simulink model "Test_Tricopter_Model"  (R2015a)
settings: Solver=ode3  SolverMode=SingleTasking  StartTime=0.0  StopTime=20  FixedStep=T_sim  RelTol=1e-3
PreLoadFcn:
  | LoadLibraries
values from neighbouring files (symbols this model uses):
  a = 10.26    [SetupComplete.m]
  A_x = 0.015    [SetupComplete.m]
  A_y = A_x    (= 0.015)    [SetupComplete.m]
  A_z = 0.16    [SetupComplete.m]
  C_d0 = 0.001193    [SetupComplete.m]
  C_x = 1.2    [SetupComplete.m]
  C_y = C_x    (= 1.2)    [SetupComplete.m]
  C_z = 2.2    [SetupComplete.m]
  CG_0 = [0,0,0.02]'    [SetupComplete.m]
  g = 9.81    [SetupComplete.m]
  h = 0.08    [SetupComplete.m]
  h_FA = 0.02    [SetupComplete.m]
  h_M = 0.064    [SetupComplete.m]
  I_BAC_0 = [ Ix,0,Ixz;0,Iy,0;Ixz,0,Iz]    [SetupComplete.m]
  I_prop = 1/4*M_eq*R^2*diag([1,1,2])    [SetupComplete.m]
  I_tube = [1/2*M_tube*R_tube_eq^2,0,  0  ;           0 ,1/3*M_tube*l_arm^2,0;             0  ,0,1/3*M_tube*l_arm^2]    [SetupComplete.m]
  Initial_Omegas = [1;1;1]*Omega_hover    [Run3Copter.m]
  J_FA = I_prop(1,1) + m_prop*h^2  + m_FA*h_FA^2 + m_M*h_M^2    [SetupComplete.m]
  J_T = J_m+1/2*M_eq*R^2    (= 2.000642e-05)    [SetupComplete.m]
  Ki = lqi(LM_4DOF_aug, Q,R)    [robust_controller.m]
  l = 0.3450    (= 0.345)    [NDI_components.m]    (also in SetupComplete.m; robust_controller.m)
  l_arm = 0.264    [SetupComplete.m]
  m = 3.51    [SetupComplete.m]
  m_0 = 2.61    [SetupComplete.m]
  m_FA = 0.02    [SetupComplete.m]
  m_M = 0.300    (= 0.3)    [SetupComplete.m]
  m_prop = 0.02    [SetupComplete.m]
  R = 0.1778    [SetupComplete.m]    (also in robust_controller.m = eye(4))
  rho = 1.15    [SetupComplete.m]
  sigma = b*c/(pi*R)    (= 0.107416159567)    [SetupComplete.m]
  T_sim = 0.01    [Run3Copter.m]
  theta_0 = 0.38397    [SetupComplete.m]
  theta_1 = -0.2967    [SetupComplete.m]
  trim_simplemodel = [0.589627915568 -2.20656039197 0 0.588313336084 0 0 0.588313330414 0 0]    [trimvalues.mat]
  V_4DOF_last = [0.0122475086001 0.00870447045314 -0.0292257707267 -0.0198753669721 -0.00290766514824 -0.0269511839788 0.0344308792695 -0.0305235710433 -0.0274078219028 -0.0329291952852 -0.0272335702183 -0.00643013158961 ... (1500 elements, 50x30)]    [NN_c_weights.mat]
  v_i0 = sqrt( 1/3*m*g/(2*rho*pi*R^2)  )    [SetupComplete.m]
  W_4DOF_last = [0.0132359246225 -0.0402459595001 -0.0221501781133 0.0046881519205 0.0457506835434 0.0464888535199 -0.0342386918322 0.0470592781761 0.0457166948243 -0.00146243512772 0.0300280468889 -0.0358113661373 ... (204 elements, 4x51)]    [NN_c_weights.mat]
undefined symbols (not defined in the file or in its folder): DOWN_0, EAST_0, Motor, NORTH_0, P_0, Prop, Q_0, R_0, sigmatest, U_0, V_0, v_i_adim, Vx_adim, Vz_adim, W_0
undefined symbols (not defined in the file): Initial_Torques, Rotation_sign, Tau_motors
libraries: simulink x61, XXCopter x32, vrlib x26, simulink_extras x6, aerolib6dofsys x3, qcatlib x3, dspinverses x3, lib_controller x2, aerolibtransform2 x2, aerolib6dof2 x1
(part 5 of 10)

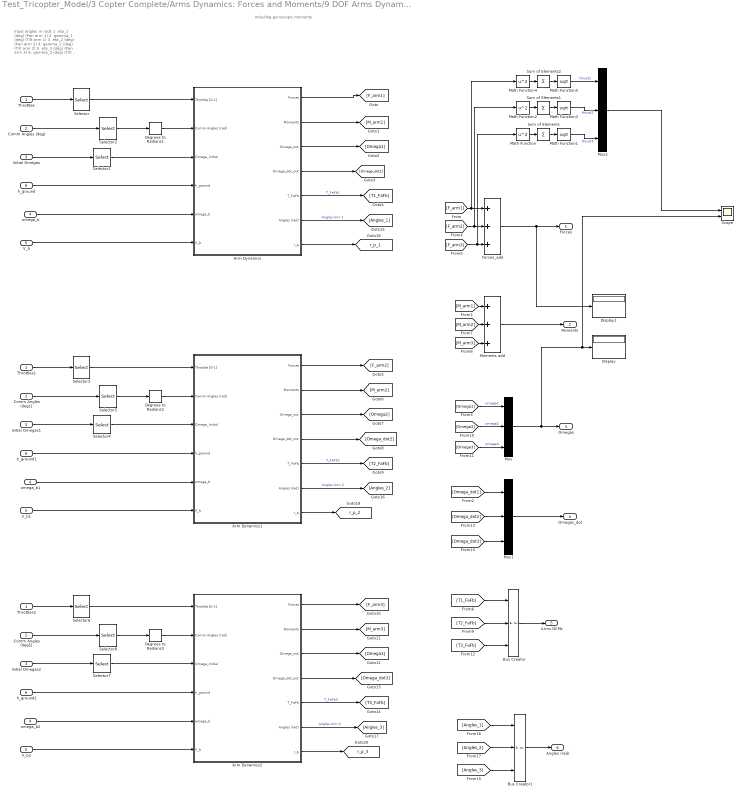
== system Test_Tricopter_Model/3 Copter Complete/Arms Dynamics: Forces and Moments/9 DOF Arms Dynamics: Forces and Moments/9 DOF Arms Dynamics: Forces and Moments ==
  note: Including gyroscopic moments
  note: Input angles in rads
      |
      | 1. eta_1 (deg)  (Pan arm 1)
      | 2. gamma_1 (deg)  (Tilt arm 1)
      |
      | 3. eta_2 (deg)  (Pan arm 2)
      | 4. gamma_2 (deg)  (Tilt arm 2)
      |
      | 5. eta_3 (deg)  (Pan arm  3)
      | 6. gamma_3 (deg)  (Tilt arm 3)
  Throttles : Inport
  Comm Angles (deg) : Inport  Port=2
  Initial Omegas : Inport  Port=3
  omega_b : Inport  Port=4
  V_b : Inport  Port=5
  h_ground : Inport  Port=6
  Arm Dynamics : Subsystem  TreatAsAtomicUnit=on  mask(Arm dynamics, kinematics, forces and moments){Rot_sign=Rotation_sign(1), tau=Tau_motors, arm_hub_pos=l*[1;0;0], arm_axis=[l_arm;0;0], arm_num=1, eta_dir=[1;0;0], gamma_dir=[0;1;0], J_T=J_T, J_FA=J_FA, h=h, Torq_ini=Initial_Torques(1), Omega_ini=Initial_Omegas(1), init_eta=0, init_gamma=0, omega_n=35, xi=1.45, c=0}
      mask prompts: Rot_sign "Rotation sign"; tau "Tau motors"; arm_hub_pos "Arm Hub position"; arm_axis "Arm Hub from servo"; arm_num "Arm number"; eta_dir "eta direcction"; gamma_dir "gamma direction"; J_T "Inertia Motor+prop"; J_FA "Inertia Forearm"; h "h propeller hub"; Torq_ini "Torque Initial Condition"; Omega_ini "Omega Initial Condition"; init_eta "Initial eta  (rad)"; init_gamma "Initial gamma  (rad)"; omega_n "Servo natural frequency"; xi "Servo damping"; c "Derivative param"
      mask help:
      | This block only accepts arms oriented in x-axis or y-axis: eta and gamma directions can only be [1,0,0] or [0,1,0]
      | Note rotations order is [eta (pan) ,gamma (tilt),0]
      |
      | If Arm number 1 (Forward one)
      | eta_dir=[1,0,0]
      | gamma_dir=[0,1,0]
      |
      | If Arm number 2 or 3 (rear ones)
      | eta_dir=[0,1,0]
      | gamma_dir=[1,0,0]
      mask TypeOptions Rot_sign: Aerodynamics Propeller/Rot_sign | Gyroscopic Moments/Rot_sign
      mask TypeOptions tau: ESC+Motor Dynamcis/tau
      mask TypeOptions arm_hub_pos: Arms Kinematics/Arm_hub_position
      mask TypeOptions arm_axis: Gyroscopic Moments/Arm_axis
      mask TypeOptions arm_num: Arms Kinematics/Arm_number
      mask TypeOptions eta_dir: Arms Kinematics/eta_dir | Gyroscopic Moments/eta_dir
      mask TypeOptions gamma_dir: Arms Kinematics/gamma_dir | Gyroscopic Moments/gamma_dir
      mask TypeOptions J_T: ESC+Motor Dynamcis/J_T | Gyroscopic Moments/J_T
      mask TypeOptions J_FA: Gyroscopic Moments/J_FA
      mask TypeOptions h: Arms Kinematics/h_prop
      mask TypeOptions Torq_ini: Initial_torque/X0
      mask TypeOptions Omega_ini: initial_omega/X0
      mask TypeOptions init_eta: Servos Dynamics/init_eta
      mask TypeOptions omega_n: Servos Dynamics/omega_n
      mask TypeOptions xi: Servos Dynamics/xi
      mask TypeOptions c: Servos Dynamics/derv_param
      mask Display:
      | % fprintf(' Arm number %i \n dynamics',arm_num)
      | 
      | 
      | disp(['{\bf \fontsize{16}',sprintf('Arm number\n\n'),num2str(arm_num),sprintf('\n\n Dynamics '),'}'], 'texmode','on');
  Arm Dynamics1 : Subsystem  TreatAsAtomicUnit=on  mask(Arm dynamics, kinematics, forces and moments){Rot_sign=Rotation_sign(2), tau=Tau_motors, arm_hub_pos=l*[-1/2;sqrt(3)/2;0], arm_axis=[0;l_arm;0], arm_num=2, eta_dir=[0;1;0], gamma_dir=[1;0;0], J_T=J_T, J_FA=J_FA, h=h, Torq_ini=Initial_Torques(2), Omega_ini=Initial_Omegas(2), init_eta=0, init_gamma=0, omega_n=35, xi=1.45, c=0}
      mask prompts: Rot_sign "Rotation sign"; tau "Tau motors"; arm_hub_pos "Arm Hub position"; arm_axis "Arm Hub from servo"; arm_num "Arm number"; eta_dir "eta direcction"; gamma_dir "gamma direction"; J_T "Inertia Motor+prop"; J_FA "Inertia Forearm"; h "h propeller hub"; Torq_ini "Torque Initial Condition"; Omega_ini "Omega Initial Condition"; init_eta "Initial eta  (rad)"; init_gamma "Initial gamma  (rad)"; omega_n "Servo natural frequency"; xi "Servo damping"; c "Derivative param"
      mask help:
      | This block only accepts arms oriented in x-axis or y-axis: eta and gamma directions can only be [1,0,0] or [0,1,0]
      | Note rotations order is [eta (pan) ,gamma (tilt),0]
      |
      | If Arm number 1 (Forward one)
      | eta_dir=[1,0,0]
      | gamma_dir=[0,1,0]
      |
      | If Arm number 2 or 3 (rear ones)
      | eta_dir=[0,1,0]
      | gamma_dir=[1,0,0]
      mask TypeOptions Rot_sign: Aerodynamics Propeller/Rot_sign | Gyroscopic Moments/Rot_sign
      mask TypeOptions tau: ESC+Motor Dynamcis/tau
      mask TypeOptions arm_hub_pos: Arms Kinematics/Arm_hub_position
      mask TypeOptions arm_axis: Gyroscopic Moments/Arm_axis
      mask TypeOptions arm_num: Arms Kinematics/Arm_number
      mask TypeOptions eta_dir: Arms Kinematics/eta_dir | Gyroscopic Moments/eta_dir
      mask TypeOptions gamma_dir: Arms Kinematics/gamma_dir | Gyroscopic Moments/gamma_dir
      mask TypeOptions J_T: ESC+Motor Dynamcis/J_T | Gyroscopic Moments/J_T
      mask TypeOptions J_FA: Gyroscopic Moments/J_FA
      mask TypeOptions h: Arms Kinematics/h_prop
      mask TypeOptions Torq_ini: Initial_torque/X0
      mask TypeOptions Omega_ini: initial_omega/X0
      mask TypeOptions init_eta: Servos Dynamics/init_eta
      mask TypeOptions omega_n: Servos Dynamics/omega_n
      mask TypeOptions xi: Servos Dynamics/xi
      mask TypeOptions c: Servos Dynamics/derv_param
      mask Display:
      | % fprintf(' Arm number %i \n dynamics',arm_num)
      | 
      | 
      | disp(['{\bf \fontsize{16}',sprintf('Arm number\n\n'),num2str(arm_num),sprintf('\n\n Dynamics '),'}'], 'texmode','on');
  Arm Dynamics2 : Subsystem  TreatAsAtomicUnit=on  mask(Arm dynamics, kinematics, forces and moments){Rot_sign=Rotation_sign(3), tau=Tau_motors, arm_hub_pos=l*[-1/2;-sqrt(3)/2;0], arm_axis=[0;-l_arm;0], arm_num=3, eta_dir=[0;1;0], gamma_dir=[1;0;0], J_T=J_T, J_FA=J_FA, h=h, Torq_ini=Initial_Torques(3), Omega_ini=Initial_Omegas(3), init_eta=0, init_gamma=0, omega_n=35, xi=1.45, c=0}
      mask prompts: Rot_sign "Rotation sign"; tau "Tau motors"; arm_hub_pos "Arm Hub position"; arm_axis "Arm Hub from servo"; arm_num "Arm number"; eta_dir "eta direcction"; gamma_dir "gamma direction"; J_T "Inertia Motor+prop"; J_FA "Inertia Forearm"; h "h propeller hub"; Torq_ini "Torque Initial Condition"; Omega_ini "Omega Initial Condition"; init_eta "Initial eta  (rad)"; init_gamma "Initial gamma  (rad)"; omega_n "Servo natural frequency"; xi "Servo damping"; c "Derivative param"
      mask help:
      | This block only accepts arms oriented in x-axis or y-axis: eta and gamma directions can only be [1,0,0] or [0,1,0]
      | Note rotations order is [eta (pan) ,gamma (tilt),0]
      |
      | If Arm number 1 (Forward one)
      | eta_dir=[1,0,0]
      | gamma_dir=[0,1,0]
      |
      | If Arm number 2 or 3 (rear ones)
      | eta_dir=[0,1,0]
      | gamma_dir=[1,0,0]
      mask TypeOptions Rot_sign: Aerodynamics Propeller/Rot_sign | Gyroscopic Moments/Rot_sign
      mask TypeOptions tau: ESC+Motor Dynamcis/tau
      mask TypeOptions arm_hub_pos: Arms Kinematics/Arm_hub_position
      mask TypeOptions arm_axis: Gyroscopic Moments/Arm_axis
      mask TypeOptions arm_num: Arms Kinematics/Arm_number
      mask TypeOptions eta_dir: Arms Kinematics/eta_dir | Gyroscopic Moments/eta_dir
      mask TypeOptions gamma_dir: Arms Kinematics/gamma_dir | Gyroscopic Moments/gamma_dir
      mask TypeOptions J_T: ESC+Motor Dynamcis/J_T | Gyroscopic Moments/J_T
      mask TypeOptions J_FA: Gyroscopic Moments/J_FA
      mask TypeOptions h: Arms Kinematics/h_prop
      mask TypeOptions Torq_ini: Initial_torque/X0
      mask TypeOptions Omega_ini: initial_omega/X0
      mask TypeOptions init_eta: Servos Dynamics/init_eta
      mask TypeOptions omega_n: Servos Dynamics/omega_n
      mask TypeOptions xi: Servos Dynamics/xi
      mask TypeOptions c: Servos Dynamics/derv_param
      mask Display:
      | % fprintf(' Arm number %i \n dynamics',arm_num)
      | 
      | 
      | disp(['{\bf \fontsize{16}',sprintf('Arm number\n\n'),num2str(arm_num),sprintf('\n\n Dynamics '),'}'], 'texmode','on');
  Bus Creator : BusCreator  Inputs=3
  Bus Creator1 : BusCreator  Inputs=3
  Comm Angles (deg)1 : InportShadow  Port=2
  Comm Angles (deg)2 : InportShadow  Port=2
  Degrees to Radians1 : simulink_extras/Transformations/Degrees to Radians
  Degrees to Radians2 : simulink_extras/Transformations/Degrees to Radians
  Degrees to Radians3 : simulink_extras/Transformations/Degrees to Radians
  Display : Display
  Display1 : Display
  Forces_add : Sum  Inputs=+++
  Initial Omegas1 : InportShadow  Port=3
  Initial Omegas2 : InportShadow  Port=3
  Math Function : Math  Operator=square  SaturateOnIntegerOverflow=on
  Math Function1 : Math  Operator=sqrt  SaturateOnIntegerOverflow=on
  Math Function2 : Math  Operator=square  SaturateOnIntegerOverflow=on
  Math Function3 : Math  Operator=sqrt  SaturateOnIntegerOverflow=on
  Math Function4 : Math  Operator=square  SaturateOnIntegerOverflow=on
  Math Function5 : Math  Operator=sqrt  SaturateOnIntegerOverflow=on
  Moments add : Sum  Inputs=+++
  Mux : Mux  Inputs=3
  Mux1 : Mux  Inputs=3
  Mux2 : Mux  Inputs=3
  Scope : Scope  NumInputPorts=2
      settings: ShowLegends=on  YMin=0~-100  YMax=17.5~700  SaveName=ScopeData4
  Selector : Selector  InputPortWidth=3  Indices=[1]
  Selector1 : Selector  InputPortWidth=3  Indices=[1]
  Selector2 : Selector  InputPortWidth=6  Indices=[1,2]
  Selector3 : Selector  InputPortWidth=3  Indices=2
  Selector4 : Selector  InputPortWidth=3  Indices=2
  Selector5 : Selector  InputPortWidth=6  Indices=[3,4]
  Selector6 : Selector  InputPortWidth=3  Indices=3
  Selector7 : Selector  InputPortWidth=3  Indices=3
  Selector8 : Selector  InputPortWidth=6  Indices=[5,6]
  Sum of Elements : Sum  Inputs=+
  Sum of Elements1 : Sum  Inputs=+
  Sum of Elements2 : Sum  Inputs=+
  Throttles1 : InportShadow
  Throttles2 : InportShadow
  V_b1 : InportShadow  Port=5
  V_b2 : InportShadow  Port=5
  h_ground1 : InportShadow  Port=6
  h_ground2 : InportShadow  Port=6
  omega_b1 : InportShadow  Port=4
  omega_b2 : InportShadow  Port=4
  Forces : Outport
  Moments : Outport  Port=2
  Omegas : Outport  Port=3
  Omegas_dot : Outport  Port=4
  Arms DCMs : Outport  Port=5
  Angles (rad) : Outport  Port=6
  tag scope: r_p_1=global, r_p_2=global, r_p_3=global
  wires:
  Selector1/1 -> Arm Dynamics/3(Omega_Initial)
  Throttles/1 -> Selector/1
  Initial Omegas/1 -> Selector1/1
  Selector/1 -> Arm Dynamics/1(Throttle [0-1])
  V_b/1 -> Arm Dynamics/6(V_b)
  Forces_add/1 -> Display1/1, Forces/1
  Moments add/1 -> Moments/1
  Mux/1 -> Scope/2, Display/1, Omegas/1
  Mux1/1 -> Omegas_dot/1
  h_ground/1 -> Arm Dynamics/4(h_ground)
  Arm Dynamics/1(Forces) -> [F_arm1]
  Arm Dynamics/2(Moments) -> [M_arm1]
  Arm Dynamics/3(Omega_out) -> [Omega1]
  Arm Dynamics/4(Omega_dot_out) -> [Omega_dot1]
  [F_arm1] -> Math Function4/1, Forces_add/1
  [M_arm1] -> Moments add/1
  [Omega_dot1] -> Mux1/1
  [Omega1] -> Mux/1  "omega1"
  omega_b/1 -> Arm Dynamics/5(omega_b)
  [F_arm2] -> Math Function2/1, Forces_add/2
  [F_arm3] -> Math Function/1, Forces_add/3
  [Omega2] -> Mux/2  "omega2"
  [Omega3] -> Mux/3  "omega3"
  [Omega_dot2] -> Mux1/2
  [Omega_dot3] -> Mux1/3
  [M_arm3] -> Moments add/3
  [M_arm2] -> Moments add/2
  Degrees to Radians1/1 -> Arm Dynamics/2(Comm Angles (rad))
  Comm Angles (deg)/1 -> Selector2/1
  Selector2/1 -> Degrees to Radians1/1
  Arm Dynamics/5(T_FaFb) -> [T1_FaFb]  "T_FaFb1"
  Bus Creator/1 -> Arms DCMs/1
  [T1_FaFb] -> Bus Creator/1
  Selector4/1 -> Arm Dynamics1/3(Omega_Initial)
  Throttles1/1 -> Selector3/1
  Initial Omegas1/1 -> Selector4/1
  Selector3/1 -> Arm Dynamics1/1(Throttle [0-1])
  V_b1/1 -> Arm Dynamics1/6(V_b)
  h_ground1/1 -> Arm Dynamics1/4(h_ground)
  Arm Dynamics1/1(Forces) -> [F_arm2]
  Arm Dynamics1/2(Moments) -> [M_arm2]
  Arm Dynamics1/3(Omega_out) -> [Omega2]
  Arm Dynamics1/4(Omega_dot_out) -> [Omega_dot2]
  omega_b1/1 -> Arm Dynamics1/5(omega_b)
  Degrees to Radians2/1 -> Arm Dynamics1/2(Comm Angles (rad))
  Comm Angles (deg)1/1 -> Selector5/1
  Selector5/1 -> Degrees to Radians2/1
  Arm Dynamics1/5(T_FaFb) -> [T2_FaFb]  "T_FaFb2"
  [T2_FaFb] -> Bus Creator/2
  Selector7/1 -> Arm Dynamics2/3(Omega_Initial)
  Throttles2/1 -> Selector6/1
  Initial Omegas2/1 -> Selector7/1
  Selector6/1 -> Arm Dynamics2/1(Throttle [0-1])
  V_b2/1 -> Arm Dynamics2/6(V_b)
  h_ground2/1 -> Arm Dynamics2/4(h_ground)
  Arm Dynamics2/1(Forces) -> [F_arm3]
  Arm Dynamics2/2(Moments) -> [M_arm3]
  Arm Dynamics2/3(Omega_out) -> [Omega3]
  Arm Dynamics2/4(Omega_dot_out) -> [Omega_dot3]
  omega_b2/1 -> Arm Dynamics2/5(omega_b)
  Degrees to Radians3/1 -> Arm Dynamics2/2(Comm Angles (rad))
  Comm Angles (deg)2/1 -> Selector8/1
  Selector8/1 -> Degrees to Radians3/1
  Arm Dynamics2/5(T_FaFb) -> [T3_FaFb]  "T_FaFb3"
  [T3_FaFb] -> Bus Creator/3
  Bus Creator1/1 -> Angles (rad)/1
  [Angles_1] -> Bus Creator1/1
  [Angles_2] -> Bus Creator1/2
  [Angles_3] -> Bus Creator1/3
  Arm Dynamics/6(Angles (rad)) -> [Angles_1]  "Angles Arm 1"
  Arm Dynamics1/6(Angles (rad)) -> [Angles_2]  "Angles Arm 2"
  Arm Dynamics2/6(Angles (rad)) -> [Angles_3]  "Angles Arm 3"
  Arm Dynamics/7(r_p) -> [r_p_1]
  Arm Dynamics1/7(r_p) -> [r_p_2]
  Arm Dynamics2/7(r_p) -> [r_p_3]
  Sum of Elements/1 -> Math Function1/1
  Math Function/1 -> Sum of Elements/1
  Sum of Elements1/1 -> Math Function3/1
  Math Function2/1 -> Sum of Elements1/1
  Math Function4/1 -> Sum of Elements2/1
  Sum of Elements2/1 -> Math Function5/1
  Math Function5/1 -> Mux2/1  "thrust1"
  Math Function3/1 -> Mux2/2  "thrust2"
  Math Function1/1 -> Mux2/3  "thrust3"
  Mux2/1 -> Scope/1

== system Test_Tricopter_Model/Controller/NDI+CA Controller/ 9DOF NDI+CA Controller - No massic update/1st order reference model ==
  y_ref : Inport
  y_meas : Inport  Port=2
  Bandwidth gain : Gain  Gain=Kb
  Bandwidth gain 1 : Gain  Gain=Kb
  Command FF gain : Gain  Gain=fc
  Command_dot FF gain : Gain  Gain=Kf
  Integral gain : Gain  Gain=fi
  Integrator : Integrator
  Integrator1 : Integrator
  Kref gain : Gain  Gain=Kref
  Sum15 : Sum  Inputs=|+-
  Sum16 : Sum  Inputs=++-
  Sum17 : Sum  Inputs=++|
  Sum5 : Sum  Inputs=|+-
  y_des_dot : Outport
  wires:
  Integral gain/1 -> Integrator1/1
  Bandwidth gain 1/1 -> Integral gain/1
  y_ref/1 -> Sum5/1
  Command_dot FF gain/1 -> Sum17/1
  Command FF gain/1 -> Sum16/1
  Integrator/1 -> Command FF gain/1, Sum15/1, Sum5/2  "y_c"
  y_meas/1 -> Sum16/3, Sum15/2
  Sum16/1 -> Bandwidth gain/1
  Kref gain/1 -> Integrator/1, Command_dot FF gain/1  "y_dot_c"
  Integrator1/1 -> Sum16/2
  Sum17/1 -> y_des_dot/1
  Bandwidth gain/1 -> Sum17/2
  Sum15/1 -> Bandwidth gain 1/1
  Sum5/1 -> Kref gain/1

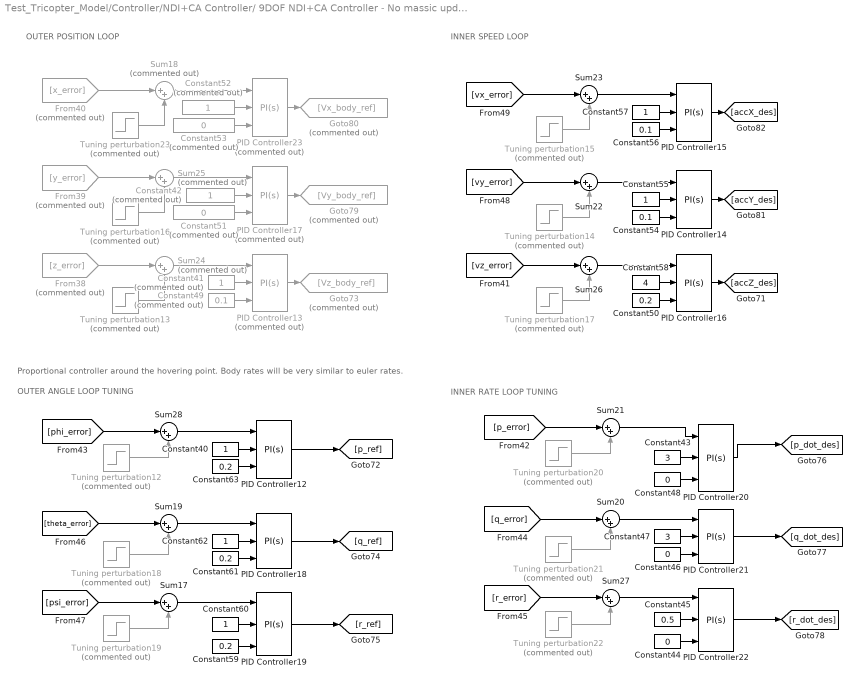
== system Test_Tricopter_Model/Controller/NDI+CA Controller/ 9DOF NDI+CA Controller - No massic update/9 DOF Ideal (Need more tuning) ==
  note: OUTER POSITION LOOP
  note: Proportional controller around the hovering point. Body rates will be very similar to euler rates.
  note: INNER RATE LOOP TUNING
  note: OUTER ANGLE LOOP TUNING
  note: INNER SPEED LOOP
  Constant{40,55,57,60,62} (5 alike) : Constant
  Constant41 : Constant  Commented=on
  Constant42 : Constant  Commented=on
  Constant43 : Constant  Value=3
  Constant44 : Constant  Value=0
  Constant45 : Constant  Value=0.5
  Constant46 : Constant  Value=0
  Constant47 : Constant  Value=3
  Constant48 : Constant  Value=0
  Constant49 : Constant  Commented=on  Value=0.1
  Constant{50,59,61,63} (4 alike) : Constant  Value=0.2
  Constant51 : Constant  Commented=on  Value=0
  Constant52 : Constant  Commented=on
  Constant53 : Constant  Commented=on  Value=0
  Constant54 : Constant  Value=0.1
  Constant56 : Constant  Value=0.1
  Constant58 : Constant  Value=4
  From38 : From  Commented=on  GotoTag=z_error
  From39 : From  Commented=on  GotoTag=y_error
  From40 : From  Commented=on  GotoTag=x_error
  Goto73 : Goto  Commented=on  GotoTag=Vz_body_ref
  Goto79 : Goto  Commented=on  GotoTag=Vy_body_ref
  Goto80 : Goto  Commented=on  GotoTag=Vx_body_ref
  PID Controller{12,14..16,18..22} (9 alike) : simulink/Continuous/PID Controller  Controller=PI  TimeDomain=Continuous-time  SampleTime=-1  IntegratorMethod=Forward Euler  FilterMethod=Forward Euler  Form=Parallel  UseFilter=on  ControllerParametersSource=external  P=1  I=1  D=0  N=100  InitialConditionSource=internal  InitialConditionForIntegrator=0  InitialConditionForFilter=0  ExternalReset=none  LimitOutput=off  UpperSaturationLimit=inf  LowerSaturationLimit=-inf  LinearizeAsGain=on  AntiWindupMode=none  Kb=1  TrackingMode=off  Kt=1  PParamMin=[]  PParamMax=[]  IParamMin=[]  IParamMax=[]  DParamMin=[]  DParamMax=[]  NParamMin=[]  NParamMax=[]  KbParamMin=[]  KbParamMax=[]  KtParamMin=[]  KtParamMax=[]  POutMin=[]  POutMax=[]  IOutMin=[]  IOutMax=[]  DOutMin=[]  DOutMax=[]  NOutMin=[]  NOutMax=[]  KbOutMin=[]  KbOutMax=[]  KtOutMin=[]  KtOutMax=[]  IntegratorOutMin=[]  IntegratorOutMax=[]  FilterOutMin=[]  FilterOutMax=[]  SumOutMin=[]  SumOutMax=[]  SumI1OutMin=[]  SumI1OutMax=[]  SumI2OutMin=[]  SumI2OutMax=[]  SumI3OutMin=[]  SumI3OutMax=[]  SumDOutMin=[]  SumDOutMax=[]  SaturationOutMin=[]  SaturationOutMax=[]  IntegratorContinuousStateAttributes=''  IntegratorStateMustResolveToSignalObject=off  IntegratorRTWStateStorageClass=Auto  FilterContinuousStateAttributes=''  FilterStateMustResolveToSignalObject=off  FilterRTWStateStorageClass=Auto  DifferentiatorICPrevScaledInput=0  DifferentiatorOutMin=[]  DifferentiatorOutMax=[]
  PID Controller13 : simulink/Continuous/PID Controller  Commented=on  Controller=PI  TimeDomain=Continuous-time  SampleTime=-1  IntegratorMethod=Forward Euler  FilterMethod=Forward Euler  Form=Parallel  UseFilter=on  ControllerParametersSource=external  P=1  I=1  D=0  N=100  InitialConditionSource=internal  InitialConditionForIntegrator=0  InitialConditionForFilter=0  ExternalReset=none  LimitOutput=off  UpperSaturationLimit=inf  LowerSaturationLimit=-inf  LinearizeAsGain=on  AntiWindupMode=none  Kb=1  TrackingMode=off  Kt=1  PParamMin=[]  PParamMax=[]  IParamMin=[]  IParamMax=[]  DParamMin=[]  DParamMax=[]  NParamMin=[]  NParamMax=[]  KbParamMin=[]  KbParamMax=[]  KtParamMin=[]  KtParamMax=[]  POutMin=[]  POutMax=[]  IOutMin=[]  IOutMax=[]  DOutMin=[]  DOutMax=[]  NOutMin=[]  NOutMax=[]  KbOutMin=[]  KbOutMax=[]  KtOutMin=[]  KtOutMax=[]  IntegratorOutMin=[]  IntegratorOutMax=[]  FilterOutMin=[]  FilterOutMax=[]  SumOutMin=[]  SumOutMax=[]  SumI1OutMin=[]  SumI1OutMax=[]  SumI2OutMin=[]  SumI2OutMax=[]  SumI3OutMin=[]  SumI3OutMax=[]  SumDOutMin=[]  SumDOutMax=[]  SaturationOutMin=[]  SaturationOutMax=[]  IntegratorContinuousStateAttributes=''  IntegratorStateMustResolveToSignalObject=off  IntegratorRTWStateStorageClass=Auto  FilterContinuousStateAttributes=''  FilterStateMustResolveToSignalObject=off  FilterRTWStateStorageClass=Auto  DifferentiatorICPrevScaledInput=0  DifferentiatorOutMin=[]  DifferentiatorOutMax=[]
  PID Controller17 : simulink/Continuous/PID Controller  Commented=on  Controller=PI  TimeDomain=Continuous-time  SampleTime=-1  IntegratorMethod=Forward Euler  FilterMethod=Forward Euler  Form=Parallel  UseFilter=on  ControllerParametersSource=external  P=1  I=1  D=0  N=100  InitialConditionSource=internal  InitialConditionForIntegrator=0  InitialConditionForFilter=0  ExternalReset=none  LimitOutput=off  UpperSaturationLimit=inf  LowerSaturationLimit=-inf  LinearizeAsGain=on  AntiWindupMode=none  Kb=1  TrackingMode=off  Kt=1  PParamMin=[]  PParamMax=[]  IParamMin=[]  IParamMax=[]  DParamMin=[]  DParamMax=[]  NParamMin=[]  NParamMax=[]  KbParamMin=[]  KbParamMax=[]  KtParamMin=[]  KtParamMax=[]  POutMin=[]  POutMax=[]  IOutMin=[]  IOutMax=[]  DOutMin=[]  DOutMax=[]  NOutMin=[]  NOutMax=[]  KbOutMin=[]  KbOutMax=[]  KtOutMin=[]  KtOutMax=[]  IntegratorOutMin=[]  IntegratorOutMax=[]  FilterOutMin=[]  FilterOutMax=[]  SumOutMin=[]  SumOutMax=[]  SumI1OutMin=[]  SumI1OutMax=[]  SumI2OutMin=[]  SumI2OutMax=[]  SumI3OutMin=[]  SumI3OutMax=[]  SumDOutMin=[]  SumDOutMax=[]  SaturationOutMin=[]  SaturationOutMax=[]  IntegratorContinuousStateAttributes=''  IntegratorStateMustResolveToSignalObject=off  IntegratorRTWStateStorageClass=Auto  FilterContinuousStateAttributes=''  FilterStateMustResolveToSignalObject=off  FilterRTWStateStorageClass=Auto  DifferentiatorICPrevScaledInput=0  DifferentiatorOutMin=[]  DifferentiatorOutMax=[]
  PID Controller23 : simulink/Continuous/PID Controller  Commented=on  Controller=PI  TimeDomain=Continuous-time  SampleTime=-1  IntegratorMethod=Forward Euler  FilterMethod=Forward Euler  Form=Parallel  UseFilter=on  ControllerParametersSource=external  P=1  I=1  D=0  N=100  InitialConditionSource=internal  InitialConditionForIntegrator=0  InitialConditionForFilter=0  ExternalReset=none  LimitOutput=off  UpperSaturationLimit=inf  LowerSaturationLimit=-inf  LinearizeAsGain=on  AntiWindupMode=none  Kb=1  TrackingMode=off  Kt=1  PParamMin=[]  PParamMax=[]  IParamMin=[]  IParamMax=[]  DParamMin=[]  DParamMax=[]  NParamMin=[]  NParamMax=[]  KbParamMin=[]  KbParamMax=[]  KtParamMin=[]  KtParamMax=[]  POutMin=[]  POutMax=[]  IOutMin=[]  IOutMax=[]  DOutMin=[]  DOutMax=[]  NOutMin=[]  NOutMax=[]  KbOutMin=[]  KbOutMax=[]  KtOutMin=[]  KtOutMax=[]  IntegratorOutMin=[]  IntegratorOutMax=[]  FilterOutMin=[]  FilterOutMax=[]  SumOutMin=[]  SumOutMax=[]  SumI1OutMin=[]  SumI1OutMax=[]  SumI2OutMin=[]  SumI2OutMax=[]  SumI3OutMin=[]  SumI3OutMax=[]  SumDOutMin=[]  SumDOutMax=[]  SaturationOutMin=[]  SaturationOutMax=[]  IntegratorContinuousStateAttributes=''  IntegratorStateMustResolveToSignalObject=off  IntegratorRTWStateStorageClass=Auto  FilterContinuousStateAttributes=''  FilterStateMustResolveToSignalObject=off  FilterRTWStateStorageClass=Auto  DifferentiatorICPrevScaledInput=0  DifferentiatorOutMin=[]  DifferentiatorOutMax=[]
  Sum{17,19..23,26..28} (9 alike) : Sum  Inputs=|++
  Sum18 : Sum  Commented=on  Inputs=|++
  Sum24 : Sum  Commented=on  Inputs=|++
  Sum25 : Sum  Commented=on  Inputs=|++
  Tuning perturbation{12,19..20,22} (4 alike) : Step  Commented=on  Time=20  After=3*pi/180  SampleTime=0
  Tuning perturbation{13..17,23} (6 alike) : Step  Commented=on  Time=20  SampleTime=0
  Tuning perturbation18 : Step  Commented=on  Time=20  After=-3*pi/180  SampleTime=0
  Tuning perturbation21 : Step  Commented=on  Time=20  After=-3*pi/180  SampleTime=0
  wires:
  Constant62/1 -> PID Controller18/2
  [vz_error] -> Sum26/1
  From38/1 -> Sum24/1
  Constant40/1 -> PID Controller12/2
  PID Controller14/1 -> [accY_des]
  [vy_error] -> Sum22/1
  Constant60/1 -> PID Controller19/2
  PID Controller15/1 -> [accX_des]
  Constant41/1 -> PID Controller13/2
  Sum23/1 -> PID Controller15/1
  Sum17/1 -> PID Controller19/1
  Constant49/1 -> PID Controller13/3
  Constant53/1 -> PID Controller23/3
  Sum18/1 -> PID Controller23/1
  Constant58/1 -> PID Controller16/2
  Tuning perturbation16/1 -> Sum25/2
  [psi_error] -> Sum17/1
  Tuning perturbation19/1 -> Sum17/2
  Sum26/1 -> PID Controller16/1
  From39/1 -> Sum25/1
  Tuning perturbation14/1 -> Sum22/2
  PID Controller13/1 -> Goto73/1
  Constant54/1 -> PID Controller14/3
  [q_error] -> Sum20/1
  Tuning perturbation23/1 -> Sum18/2
  Constant52/1 -> PID Controller23/2
  Sum20/1 -> PID Controller21/1
  From40/1 -> Sum18/1
  Tuning perturbation18/1 -> Sum19/2
  Constant61/1 -> PID Controller18/3
  Constant50/1 -> PID Controller16/3
  Tuning perturbation12/1 -> Sum28/2
  Constant44/1 -> PID Controller22/3
  Constant46/1 -> PID Controller21/3
  Tuning perturbation15/1 -> Sum23/2
  Tuning perturbation22/1 -> Sum27/2
  PID Controller12/1 -> [p_ref]
  Sum21/1 -> PID Controller20/1
  Constant43/1 -> PID Controller20/2
  Sum25/1 -> PID Controller17/1
  PID Controller18/1 -> [q_ref]
  Tuning perturbation13/1 -> Sum24/2
  Sum27/1 -> PID Controller22/1
  Constant56/1 -> PID Controller15/3
  Sum19/1 -> PID Controller18/1
  PID Controller23/1 -> Goto80/1
  Sum24/1 -> PID Controller13/1
  PID Controller17/1 -> Goto79/1
  PID Controller20/1 -> [p_dot_des]
  [r_error] -> Sum27/1
  [phi_error] -> Sum28/1
  [vx_error] -> Sum23/1
  PID Controller16/1 -> [accZ_des]
  Sum28/1 -> PID Controller12/1
  Constant47/1 -> PID Controller21/2
  [p_error] -> Sum21/1
  Sum22/1 -> PID Controller14/1
  Tuning perturbation17/1 -> Sum26/2
  Constant63/1 -> PID Controller12/3
  PID Controller21/1 -> [q_dot_des]
  Constant51/1 -> PID Controller17/3
  Tuning perturbation21/1 -> Sum20/2
  Constant45/1 -> PID Controller22/2
  Constant42/1 -> PID Controller17/2
  PID Controller19/1 -> [r_ref]
  Constant59/1 -> PID Controller19/3
  Constant55/1 -> PID Controller14/2
  [theta_error] -> Sum19/1
  PID Controller22/1 -> [r_dot_des]
  Tuning perturbation20/1 -> Sum21/2
  Constant57/1 -> PID Controller15/2
  Constant48/1 -> PID Controller20/3

== system Test_Tricopter_Model/Controller/NDI+CA Controller/ 9DOF NDI+CA Controller - No massic update/Control Allocation 9DOF ==
  Pseudocontrol input : Inport
  Effectiveness control matrix : Inport  Port=2
  Control Allocation 9DOF : Subsystem  VariantControl=(default)
  Pseudoinverse 9DOF : Subsystem  VariantControl=Variant1
  Control output : Outport

== system Test_Tricopter_Model/Controller/NDI+CA Controller/4DOF ANN+NDI+CA Controller - No massic update/Adaptive NN ==
  Model Reference Vars : Inport
  System State Vars : Inport  Port=2
  v_ad^ prev : Inport  Port=3
  Crossed NN : Subsystem  VariantControl=NN on AoA
  v_ad^ : Outport

== system Test_Tricopter_Model/Controller/NDI+CA Controller/4DOF ANN+NDI+CA Controller - No massic update/Control Allocation 4DOF ==
  Pseudocontrol input : Inport
  Effectiveness control matrix : Inport  Port=2
  Control Allocation 4DOF : Subsystem  VariantControl=(default)
  Pseudoinverse : Subsystem  VariantControl=Variant1
  Control output : Outport

== system Test_Tricopter_Model/Controller/NDI+CA Controller/4DOF ANN+NDI+CA Controller - No massic update/Measurement noise ==
  Measurement : Inport
  Activate : Inport  Port=2
  Mux : Mux  Inputs=3
  Product : Product
  Random Number : RandomNumber  Variance=sigma_noise  SampleTime=0.1
  Random Number1 : RandomNumber  Variance=sigma_noise  SampleTime=0.1
  Random Number2 : RandomNumber  Variance=sigma_noise  SampleTime=0.1
  Scope : Scope
      settings: YMin=-0.2  YMax=0.2  SaveName=ScopeData16
  Sum : Sum  Inputs=|++
  Noisy Output : Outport
  wires:
  Measurement/1 -> Sum/1
  Random Number/1 -> Mux/1
  Random Number1/1 -> Mux/2
  Random Number2/1 -> Mux/3
  Mux/1 -> Scope/1, Product/2
  Activate/1 -> Product/1
  Product/1 -> Sum/2
  Sum/1 -> Noisy Output/1

== system Test_Tricopter_Model/Controller/NDI+CA Controller/4DOF ANN+NDI+CA Controller - No massic update/Phi Model Reference ==
  u_ref : Inport
  y_dot : Inport  Port=2
  y : Inport  Port=3
  pch : Inport  Port=4
  A_error_dynamics : Constant  Value=[0, 1; -(r*omega_n)^2, -2*xi*(r*omega_n)]
  Bus Creator : BusCreator  Inputs=8
  Kd_y_dot : Gain  Gain=2*xi*(r*omega_n)
  Kp_y : Gain  Gain=(r*omega_n)^2
  P_error_dynamics : Constant  Value=[((r*omega_n)^2+1)/(2*xi*(r*omega_n)) + 2*xi*(r*omega_n)/(r*omega_n)^2, 1/(r*omega_n)^2; 1/(r*omega_n)^2, (1+1/(r*omega_n)^2)/(2*xi*(r*omega_n))]
  Reference Model1 : Subsystem  AncestorBlock=Adaptive_FaultTolerantControl/Ref Model and P Controller/Reference Model  mask{omega_n=omega_n, xi=xi}
      mask prompts: omega_n "Natural Frequency"; xi "Damping"
      mask help:
      | 2nd Order System
      | Only provides output acceleration
      mask Display:
      | TF = tf([omega_n^2],[1 2*xi*omega_n omega_n^2]);
      | 
      | [y,t]=step(TF);
      | S = stepinfo(y,t);
      | 
      | pos = get_param(gcb, 'Position');
      | width = pos(3) - pos(1);
      | height = pos(4) - pos(2);
      | t = t.*width/max(t);
      | y=y.*height/max(y);
      | plot(t,y);
      | S2 = stepinfo(y,t);
      | 
      | if S.Overshoot==0 % 1st order response
      |     text(S2.RiseTime ,height*0.85,['Rise time = ',num2str(S.RiseTime),'s' ]);
      |     text(S2.RiseTime ,height*0.75,['Settling Time = ',num2str(S.SettlingTime)]);
      | 
      | elseif S.Overshoot<0.05 % 2nd order response
      |     text(width*0.5 ,height*0.9,['Rise time = ',num2str(S.RiseTime),'s' ]);
      |     text(width*0.5 ,height*0.8,['Pike time = ',num2str(S.PeakTime),'s' ]);
      |     text(width*0.5 ,height*0.7,['Os = ',num2str(S.Peak)]);
      |     text(width*0.5 ,height*0.6,['SettlingTime = ',num2str(S.SettlingTime)]);
      | else % 2nd order response
      |     text(S2.PeakTime ,S2.Peak*0.85,['Peak time = ',num2str(S.PeakTime),'s' ]);
      |     text(S2.PeakTime ,S2.Peak*0.75,['Os = ',num2str(S.Peak)]);
      |     text(S2.PeakTime ,S2.Peak*0.65,['SettlingTime = ',num2str(S.SettlingTime)]);
      | end
      | 
      | 
      | [num,den] = tfdata(TF);
      | dpoly(num{:},den{:}, 's');
  Sum19 : Sum  Inputs=|+-
  Sum20 : Sum  Inputs=+++
  Sum21 : Sum  Inputs=|+-
  b_error_dynamics : Constant  Value=[0; 1]  VectorParams1D=off
  y_dot_dot_des : Outport
  NN_variables : Outport  Port=2
  wires:
  Reference Model1/1(y_dot_dot) -> Bus Creator/5, Sum20/1  "y_dot_dot_c"
  Reference Model1/3(y) -> Bus Creator/3, Sum19/1  "y_c"
  u_ref/1 -> Reference Model1/1(u)
  y/1 -> Sum19/2
  Sum19/1 -> Bus Creator/1, Kp_y/1  "y_error"
  Reference Model1/2(y_dot) -> Bus Creator/4, Sum21/1  "y_dot_c"
  y_dot/1 -> Sum21/2
  Sum21/1 -> Bus Creator/2, Kd_y_dot/1  "y_dot_error"
  Kp_y/1 -> Sum20/3
  Kd_y_dot/1 -> Sum20/2
  Sum20/1 -> y_dot_dot_des/1
  Bus Creator/1 -> NN_variables/1
  P_error_dynamics/1 -> Bus Creator/6  "P_error_dyn"
  A_error_dynamics/1 -> Bus Creator/7  "A_error_dyn"
  b_error_dynamics/1 -> Bus Creator/8  "b_error_dyn"
  pch/1 -> Reference Model1/2(pch)

== system Test_Tricopter_Model/Controller/NDI+CA Controller/4DOF ANN+NDI+CA Controller - No massic update/Sigmoid  ==
  In : Inport
  Display : Display
  Fcn1 : Fcn  Commented=on  Expr=2.0 ./ (1.0 + exp(-u(4)*u(1:3)))-1
  MATLAB Function : MATLAB Function  TreatAsAtomicUnit=on
  a : Constant  Value=a
  Out : Outport
  wires:
  MATLAB Function/1(y) -> Display/1, Out/1
  In/1 -> MATLAB Function/1(u)
  a/1 -> MATLAB Function/2(a)

== system Test_Tricopter_Model/Controller/NDI+CA Controller/4DOF ANN+NDI+CA Controller - No massic update/Theta Model Reference1 ==
  u_ref : Inport
  y_dot : Inport  Port=2
  y : Inport  Port=3
  pch : Inport  Port=4
  A_error_dynamics1 : Constant  Value=[0, 1; -(r*omega_n)^2, -2*xi*(r*omega_n)]
  Bus Creator : BusCreator  Inputs=8
  Kd_y_dot : Gain  Gain=2*xi*(r*omega_n)
  Kp_y : Gain  Gain=(r*omega_n)^2
  P_error_dynamics1 : Constant  Value=[((r*omega_n)^2+1)/(2*xi*(r*omega_n)) + 2*xi*(r*omega_n)/(r*omega_n)^2, 1/(r*omega_n)^2; 1/(r*omega_n)^2, (1+1/(r*omega_n)^2)/(2*xi*(r*omega_n))]
  Reference Model1 : Subsystem  AncestorBlock=Adaptive_FaultTolerantControl/Ref Model and P Controller/Reference Model  mask{omega_n=omega_n, xi=xi}
      mask prompts: omega_n "Natural Frequency"; xi "Damping"
      mask help:
      | 2nd Order System
      | Only provides output acceleration
      mask Display:
      | TF = tf([omega_n^2],[1 2*xi*omega_n omega_n^2]);
      | 
      | [y,t]=step(TF);
      | S = stepinfo(y,t);
      | 
      | pos = get_param(gcb, 'Position');
      | width = pos(3) - pos(1);
      | height = pos(4) - pos(2);
      | t = t.*width/max(t);
      | y=y.*height/max(y);
      | plot(t,y);
      | S2 = stepinfo(y,t);
      | 
      | if S.Overshoot==0 % 1st order response
      |     text(S2.RiseTime ,height*0.85,['Rise time = ',num2str(S.RiseTime),'s' ]);
      |     text(S2.RiseTime ,height*0.75,['Settling Time = ',num2str(S.SettlingTime)]);
      | 
      | elseif S.Overshoot<0.05 % 2nd order response
      |     text(width*0.5 ,height*0.9,['Rise time = ',num2str(S.RiseTime),'s' ]);
      |     text(width*0.5 ,height*0.8,['Pike time = ',num2str(S.PeakTime),'s' ]);
      |     text(width*0.5 ,height*0.7,['Os = ',num2str(S.Peak)]);
      |     text(width*0.5 ,height*0.6,['SettlingTime = ',num2str(S.SettlingTime)]);
      | else % 2nd order response
      |     text(S2.PeakTime ,S2.Peak*0.85,['Peak time = ',num2str(S.PeakTime),'s' ]);
      |     text(S2.PeakTime ,S2.Peak*0.75,['Os = ',num2str(S.Peak)]);
      |     text(S2.PeakTime ,S2.Peak*0.65,['SettlingTime = ',num2str(S.SettlingTime)]);
      | end
      | 
      | 
      | [num,den] = tfdata(TF);
      | dpoly(num{:},den{:}, 's');
  Sum19 : Sum  Inputs=|+-
  Sum20 : Sum  Inputs=+++
  Sum21 : Sum  Inputs=|+-
  b_error_dynamics : Constant  Value=[0; 1]  VectorParams1D=off
  y_dot_dot_des : Outport
  NN_variables : Outport  Port=2
  wires:
  b_error_dynamics/1 -> Bus Creator/8  "b_error_dyn"
  A_error_dynamics1/1 -> Bus Creator/7  "A_error_dyn"
  P_error_dynamics1/1 -> Bus Creator/6  "P_error_dyn"
  Bus Creator/1 -> NN_variables/1
  Sum20/1 -> y_dot_dot_des/1
  Kd_y_dot/1 -> Sum20/2
  Kp_y/1 -> Sum20/3
  Sum21/1 -> Bus Creator/2, Kd_y_dot/1  "y_dot_error"
  y_dot/1 -> Sum21/2
  Reference Model1/2(y_dot) -> Sum21/1, Bus Creator/4  "y_dot_c"
  Sum19/1 -> Kp_y/1, Bus Creator/1  "y_error"
  y/1 -> Sum19/2
  u_ref/1 -> Reference Model1/1(u)
  Reference Model1/3(y) -> Sum19/1, Bus Creator/3  "y_c"
  Reference Model1/1(y_dot_dot) -> Sum20/1, Bus Creator/5  "y_dot_dot_c"
  pch/1 -> Reference Model1/2(pch)

== system Test_Tricopter_Model/Controller/NDI+CA Controller/4DOF NDI+CA Controller - No massic update/1st order reference model ==
  y_ref : Inport
  y_meas : Inport  Port=2
  Bandwidth gain : Gain  Gain=Kb
  Bandwidth gain 1 : Gain  Gain=Kb
  Command FF gain : Gain  Gain=fc
  Command_dot FF gain : Gain  Gain=Kf
  Integral gain : Gain  Gain=fi
  Integrator : Integrator
  Integrator1 : Integrator
  Kref gain : Gain  Gain=Kref
  Sum15 : Sum  Inputs=|+-
  Sum16 : Sum  Inputs=++-
  Sum17 : Sum  Inputs=++|
  Sum5 : Sum  Inputs=|+-
  y_des_dot : Outport
  wires:
  Integral gain/1 -> Integrator1/1
  Bandwidth gain 1/1 -> Integral gain/1
  y_ref/1 -> Sum5/1
  Command_dot FF gain/1 -> Sum17/1
  Command FF gain/1 -> Sum16/1
  Integrator/1 -> Command FF gain/1, Sum15/1, Sum5/2  "y_c"
  y_meas/1 -> Sum16/3, Sum15/2
  Sum16/1 -> Bandwidth gain/1
  Kref gain/1 -> Integrator/1, Command_dot FF gain/1  "y_dot_c"
  Integrator1/1 -> Sum16/2
  Sum17/1 -> y_des_dot/1
  Bandwidth gain/1 -> Sum17/2
  Sum15/1 -> Bandwidth gain 1/1
  Sum5/1 -> Kref gain/1

== system Test_Tricopter_Model/Controller/NDI+CA Controller/4DOF NDI+CA Controller - No massic update/1st order reference model1 ==
  y_ref : Inport
  y_meas : Inport  Port=2
  Bandwidth gain : Gain  Gain=Kb
  Bandwidth gain 1 : Gain  Gain=Kb
  Command FF gain : Gain  Gain=fc
  Command_dot FF gain : Gain  Gain=Kf
  Integral gain : Gain  Gain=fi
  Integrator : Integrator
  Integrator1 : Integrator
  Kref gain : Gain  Gain=Kref
  Sum15 : Sum  Inputs=|+-
  Sum16 : Sum  Inputs=++-
  Sum17 : Sum  Inputs=++|
  Sum5 : Sum  Inputs=|+-
  y_des_dot : Outport
  wires:
  Sum5/1 -> Kref gain/1
  Sum15/1 -> Bandwidth gain 1/1
  Bandwidth gain/1 -> Sum17/2
  Sum17/1 -> y_des_dot/1
  Integrator1/1 -> Sum16/2
  Kref gain/1 -> Command_dot FF gain/1, Integrator/1  "y_dot_c"
  Sum16/1 -> Bandwidth gain/1
  y_meas/1 -> Sum15/2, Sum16/3
  Integrator/1 -> Sum5/2, Sum15/1, Command FF gain/1  "y_c"
  Command FF gain/1 -> Sum16/1
  Command_dot FF gain/1 -> Sum17/1
  y_ref/1 -> Sum5/1
  Bandwidth gain 1/1 -> Integral gain/1
  Integral gain/1 -> Integrator1/1

== system Test_Tricopter_Model/Controller/NDI+CA Controller/4DOF NDI+CA Controller - No massic update/1st order reference model2 ==
  y_ref : Inport
  y_meas : Inport  Port=2
  Bandwidth gain : Gain  Gain=Kb
  Bandwidth gain 1 : Gain  Gain=Kb
  Command FF gain : Gain  Gain=fc
  Command_dot FF gain : Gain  Gain=Kf
  Integral gain : Gain  Gain=fi
  Integrator : Integrator
  Integrator1 : Integrator
  Kref gain : Gain  Gain=Kref
  Sum15 : Sum  Inputs=|+-
  Sum16 : Sum  Inputs=++-
  Sum17 : Sum  Inputs=++|
  Sum5 : Sum  Inputs=|+-
  y_des_dot : Outport
  wires:
  Integral gain/1 -> Integrator1/1
  Bandwidth gain 1/1 -> Integral gain/1
  y_ref/1 -> Sum5/1
  Command_dot FF gain/1 -> Sum17/1
  Command FF gain/1 -> Sum16/1
  Integrator/1 -> Command FF gain/1, Sum15/1, Sum5/2  "y_c"
  y_meas/1 -> Sum16/3, Sum15/2
  Sum16/1 -> Bandwidth gain/1
  Kref gain/1 -> Integrator/1, Command_dot FF gain/1  "y_dot_c"
  Integrator1/1 -> Sum16/2
  Sum17/1 -> y_des_dot/1
  Bandwidth gain/1 -> Sum17/2
  Sum15/1 -> Bandwidth gain 1/1
  Sum5/1 -> Kref gain/1

== system Test_Tricopter_Model/Controller/NDI+CA Controller/4DOF NDI+CA Controller - No massic update/1st order reference model3 ==
  y_ref : Inport
  y_meas : Inport  Port=2
  Bandwidth gain : Gain  Gain=Kb
  Bandwidth gain 1 : Gain  Gain=Kb
  Command FF gain : Gain  Gain=fc
  Command_dot FF gain : Gain  Gain=Kf
  Integral gain : Gain  Gain=fi
  Integrator : Integrator
  Integrator1 : Integrator
  Kref gain : Gain  Gain=Kref
  Sum15 : Sum  Inputs=|+-
  Sum16 : Sum  Inputs=++-
  Sum17 : Sum  Inputs=++|
  Sum5 : Sum  Inputs=|+-
  y_des_dot : Outport
  wires:
  Sum5/1 -> Kref gain/1
  Sum15/1 -> Bandwidth gain 1/1
  Bandwidth gain/1 -> Sum17/2
  Sum17/1 -> y_des_dot/1
  Integrator1/1 -> Sum16/2
  Kref gain/1 -> Command_dot FF gain/1, Integrator/1  "y_dot_c"
  Sum16/1 -> Bandwidth gain/1
  y_meas/1 -> Sum15/2, Sum16/3
  Integrator/1 -> Sum5/2, Sum15/1, Command FF gain/1  "y_c"
  Command FF gain/1 -> Sum16/1
  Command_dot FF gain/1 -> Sum17/1
  y_ref/1 -> Sum5/1
  Bandwidth gain 1/1 -> Integral gain/1
  Integral gain/1 -> Integrator1/1

== system Test_Tricopter_Model/Controller/NDI+CA Controller/4DOF NDI+CA Controller - No massic update/1st order reference model4 ==
  y_ref : Inport
  y_meas : Inport  Port=2
  Bandwidth gain : Gain  Gain=Kb
  Bandwidth gain 1 : Gain  Gain=Kb
  Command FF gain : Gain  Gain=fc
  Command_dot FF gain : Gain  Gain=Kf
  Integral gain : Gain  Gain=fi
  Integrator : Integrator
  Integrator1 : Integrator
  Kref gain : Gain  Gain=Kref
  Sum15 : Sum  Inputs=|+-
  Sum16 : Sum  Inputs=++-
  Sum17 : Sum  Inputs=++|
  Sum5 : Sum  Inputs=|+-
  y_des_dot : Outport
  wires:
  Integral gain/1 -> Integrator1/1
  Bandwidth gain 1/1 -> Integral gain/1
  y_ref/1 -> Sum5/1
  Command_dot FF gain/1 -> Sum17/1
  Command FF gain/1 -> Sum16/1
  Integrator/1 -> Command FF gain/1, Sum15/1, Sum5/2  "y_c"
  y_meas/1 -> Sum16/3, Sum15/2
  Sum16/1 -> Bandwidth gain/1
  Kref gain/1 -> Integrator/1, Command_dot FF gain/1  "y_dot_c"
  Integrator1/1 -> Sum16/2
  Sum17/1 -> y_des_dot/1
  Bandwidth gain/1 -> Sum17/2
  Sum15/1 -> Bandwidth gain 1/1
  Sum5/1 -> Kref gain/1

== system Test_Tricopter_Model/Controller/NDI+CA Controller/4DOF NDI+CA Controller - No massic update/1st order reference model5 ==
  y_ref : Inport
  y_meas : Inport  Port=2
  Bandwidth gain : Gain  Gain=Kb
  Bandwidth gain 1 : Gain  Gain=Kb
  Command FF gain : Gain  Gain=fc
  Command_dot FF gain : Gain  Gain=Kf
  Integral gain : Gain  Gain=fi
  Integrator : Integrator
  Integrator1 : Integrator
  Kref gain : Gain  Gain=Kref
  Sum15 : Sum  Inputs=|+-
  Sum16 : Sum  Inputs=++-
  Sum17 : Sum  Inputs=++|
  Sum5 : Sum  Inputs=|+-
  y_des_dot : Outport
  wires:
  Sum5/1 -> Kref gain/1
  Sum15/1 -> Bandwidth gain 1/1
  Bandwidth gain/1 -> Sum17/2
  Sum17/1 -> y_des_dot/1
  Integrator1/1 -> Sum16/2
  Kref gain/1 -> Command_dot FF gain/1, Integrator/1  "y_dot_c"
  Sum16/1 -> Bandwidth gain/1
  y_meas/1 -> Sum15/2, Sum16/3
  Integrator/1 -> Sum5/2, Sum15/1, Command FF gain/1  "y_c"
  Command FF gain/1 -> Sum16/1
  Command_dot FF gain/1 -> Sum17/1
  y_ref/1 -> Sum5/1
  Bandwidth gain 1/1 -> Integral gain/1
  Integral gain/1 -> Integrator1/1

== system Test_Tricopter_Model/Controller/NDI+CA Controller/4DOF NDI+CA Controller - No massic update/1st order reference model6 ==
  y_ref : Inport
  y_meas : Inport  Port=2
  Bandwidth gain : Gain  Gain=Kb
  Bandwidth gain 1 : Gain  Gain=Kb
  Command FF gain : Gain  Gain=fc
  Command_dot FF gain : Gain  Gain=Kf
  Integral gain : Gain  Gain=fi
  Integrator : Integrator
  Integrator1 : Integrator
  Kref gain : Gain  Gain=Kref
  Sum15 : Sum  Inputs=|+-
  Sum16 : Sum  Inputs=++-
  Sum17 : Sum  Inputs=++|
  Sum5 : Sum  Inputs=|+-
  y_des_dot : Outport
  wires:
  Integral gain/1 -> Integrator1/1
  Bandwidth gain 1/1 -> Integral gain/1
  y_ref/1 -> Sum5/1
  Command_dot FF gain/1 -> Sum17/1
  Command FF gain/1 -> Sum16/1
  Integrator/1 -> Command FF gain/1, Sum15/1, Sum5/2  "y_c"
  y_meas/1 -> Sum16/3, Sum15/2
  Sum16/1 -> Bandwidth gain/1
  Kref gain/1 -> Integrator/1, Command_dot FF gain/1  "y_dot_c"
  Integrator1/1 -> Sum16/2
  Sum17/1 -> y_des_dot/1
  Bandwidth gain/1 -> Sum17/2
  Sum15/1 -> Bandwidth gain 1/1
  Sum5/1 -> Kref gain/1

== system Test_Tricopter_Model/Controller/NDI+CA Controller/4DOF NDI+CA Controller - No massic update/1st order reference model7 ==
  y_ref : Inport
  y_meas : Inport  Port=2
  Bandwidth gain : Gain  Gain=Kb
  Bandwidth gain 1 : Gain  Gain=Kb
  Command FF gain : Gain  Gain=fc
  Command_dot FF gain : Gain  Gain=Kf
  Integral gain : Gain  Gain=fi
  Integrator : Integrator
  Integrator1 : Integrator
  Kref gain : Gain  Gain=Kref
  Sum15 : Sum  Inputs=|+-
  Sum16 : Sum  Inputs=++-
  Sum17 : Sum  Inputs=++|
  Sum5 : Sum  Inputs=|+-
  y_des_dot : Outport
  wires:
  Sum5/1 -> Kref gain/1
  Sum15/1 -> Bandwidth gain 1/1
  Bandwidth gain/1 -> Sum17/2
  Sum17/1 -> y_des_dot/1
  Integrator1/1 -> Sum16/2
  Kref gain/1 -> Command_dot FF gain/1, Integrator/1  "y_dot_c"
  Sum16/1 -> Bandwidth gain/1
  y_meas/1 -> Sum15/2, Sum16/3
  Integrator/1 -> Sum5/2, Sum15/1, Command FF gain/1  "y_c"
  Command FF gain/1 -> Sum16/1
  Command_dot FF gain/1 -> Sum17/1
  y_ref/1 -> Sum5/1
  Bandwidth gain 1/1 -> Integral gain/1
  Integral gain/1 -> Integrator1/1

== system Test_Tricopter_Model/Controller/NDI+CA Controller/4DOF NDI+CA Controller - No massic update/Control Allocation 4DOF ==
  Pseudocontrol input : Inport
  Effectiveness control matrix : Inport  Port=2
  Control Allocation 4DOF : Subsystem  VariantControl=(default)
  Pseudoinverse : Subsystem  VariantControl=Variant1
  Control output : Outport
